simulink model "double_pend_sim"  (R2017b)
settings: Solver=VariableStepAuto  StartTime=0.0  StopTime=10.0  RelTol=1e-3
settings Model: Creator=ozhanyz  LastModifiedBy=ozhanyz

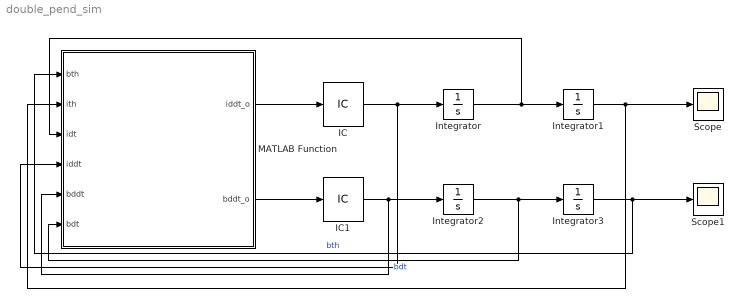
== system double_pend_sim ==
  IC : InitialCondition  Value=0.0000001
  IC1 : InitialCondition  Value=0.0000001
  Integrator : Integrator
  Integrator1 : Integrator  InitialCondition=0.994
  Integrator2 : Integrator
  Integrator3 : Integrator  InitialCondition=-0.366
  MATLAB Function : MATLAB Function  TreatAsAtomicUnit=on
  Scope : Scope
  Scope1 : Scope
  wires:
  Integrator/1 -> MATLAB Function/3(idt), Integrator1/1
  Integrator1/1 -> MATLAB Function/2(ith), Scope/1
  IC/1 -> MATLAB Function/4(iddt), Integrator/1
  IC1/1 -> MATLAB Function/5(bddt), Integrator2/1
  Integrator3/1 -> MATLAB Function/1(bth), Scope1/1  "bth"
  Integrator2/1 -> MATLAB Function/6(bdt), Integrator3/1  "bdt"
  MATLAB Function/1(iddt_o) -> IC/1
  MATLAB Function/2(bddt_o) -> IC1/1

== matlab function double_pend_sim/MATLAB Function ==
  data: bth input; iddt_o output; ith input; idt input; iddt input; bddt input; bdt input; bddt_o output
function [iddt_o,bddt_o] = double_pend_sim(bth,ith,idt,iddt,bddt,bdt)
m=2;
l=1;
g=9.81;
k=5;

M=m*g*l/(2*m*l*l);
K=k/(m*l*l);

iddt_o=3*(((idt^2)*sin(ith-bth)/4)-(iddt*cos(ith-bth)/4)-2*K*bth+K*ith+3*M*sin(bth))/4;
bddt_o=3*((-bddt^2*cos(ith-bth)/4)-(bdt^2*sin(ith-bth)/4)-K*(ith-bth)+M*sin(ith));
